simulink model "ArduCopter"  (R2016a)
settings: Solver=ode8  SolverMode=SingleTasking  StartTime=0.0  StopTime=endtime_selfdefine  FixedStep=0.0025  RelTol=1e-3
InitFcn:
  | %load QuadCopterParameters
values from neighbouring files (symbols this model uses):
  Discretetime_400Hz = 0.0025    [euler_roll_angle_cd.mat]
  flight_mode = 1    [flight_control_run.m]
undefined symbols (not defined in the file or in its folder): Cutoff_frequency_acc_z, D_acc_z, D_vel_x, D_vel_y, DEG_TO_RAD, Discretetime_1Hz, g, I_acc_z, I_vel_x, I_vel_y, Kp_angle, MotorLayout, P_acc_z, P_pos_x, P_pos_y, P_pos_z, P_vel_x, P_vel_y, P_vel_z, thrust_rpyt_down, thrust_rpyt_up
libraries: Lib_AC_AttitudeControl x26, Lib_AP_Math x26, Lib_AP_Motors x5, Lib_AC_PID x4, Lib_AP_AHRS x3, simulink x1
(part 1 of 2)
settings Model: Creator=Ehang  LastModifiedBy=Administrator
settings DataIOCC: LimitDataPoints=on  SaveFormat=Array  SaveOutput=off  SaveTime=off
settings DebuggingCC: SignalInfNanChecking=error  SolverPrmCheckMsg=warning  InheritedTsInSrcMsg=none  UnconnectedInputMsg=none  UnconnectedOutputMsg=none  UnconnectedLineMsg=none
settings HardwareCC: ProdBitPerPointer=32  ProdLargestAtomicFloat=None  ProdIntDivRoundTo=Undefined  ProdEndianess=Unspecified  ProdWordSize=32  ProdHWDeviceType=32-bit Generic
settings ModelReferenceCC: ModelReferenceNumInstancesAllowed=Single  PropagateSignalLabelsOutOfModel=off
settings GRTTargetCC: MatFileLogging=off
settings ConfigComp: CovModelRefEnable=Off  CovSFcnEnable=off

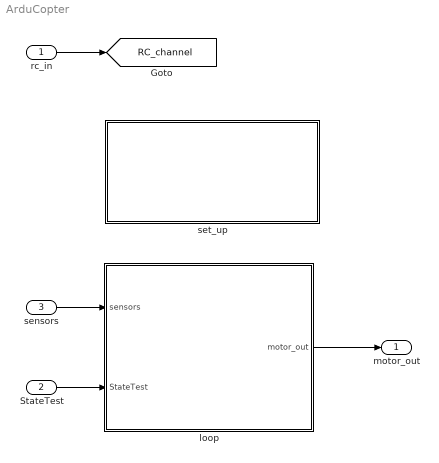
== system ArduCopter ==
  rc_in : Inport  PortDimensions=channelnum
  StateTest : Inport  Port=2  OutDataTypeStr=Bus: VehicleStates
  sensors : Inport  Port=3  OutDataTypeStr=Bus: Sensors
  loop : Subsystem
  set_up : Subsystem  Description=AC_PID控制库
  motor_out : Outport
  tag scope: RC_channel=global
  wires:
  rc_in/1 -> [RC_channel]
  loop/1(motor_out) -> motor_out/1
  sensors/1 -> loop/1(sensors)
  StateTest/1 -> loop/2(StateTest)

== system ArduCopter/loop ==
  sensors : Inport  OutDataTypeStr=Bus: Sensors
  StateTest : Inport  Port=2  OutDataTypeStr=Bus: VehicleStates
  LogData : Subsystem
  Slow-to-Fast Transition1 : RateTransition  OutPortSampleTime=0.0025
  fast_loop : Subsystem
  motors_trysignal : Constant
  scheduler.run : Subsystem  Description=AC_PID控制库
  motor_out : Outport
  wires:
  motors_trysignal/1 -> scheduler.run/1(motors_flag)
  scheduler.run/1(MortorMatix) -> Slow-to-Fast Transition1/1
  Slow-to-Fast Transition1/1 -> fast_loop/3(MotorMatix)
  fast_loop/1(motor_out) -> motor_out/1
  sensors/1 -> fast_loop/1(sensors)
  StateTest/1 -> fast_loop/2(StateTest)

== system ArduCopter/set_up ==

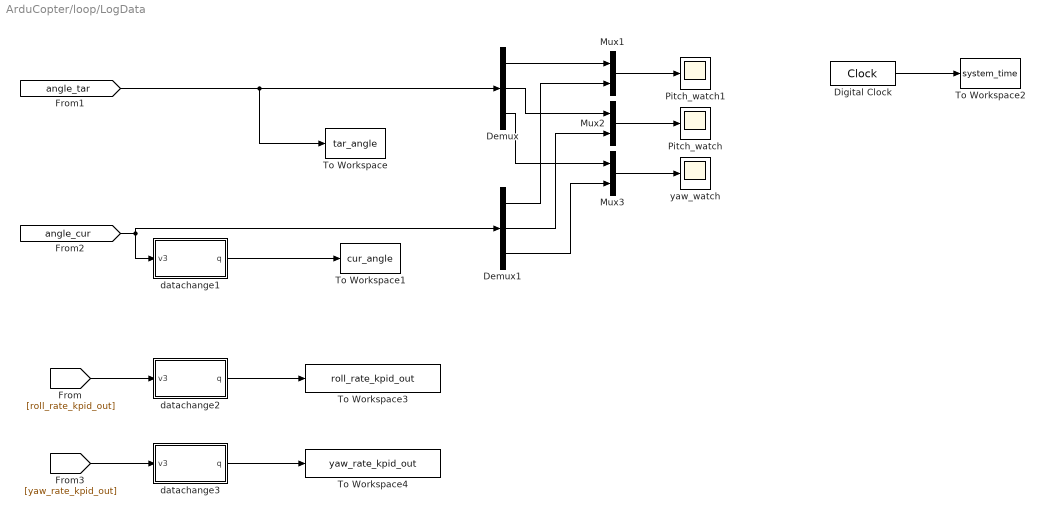
== system ArduCopter/loop/LogData ==
  Demux : Demux  Outputs=3
  Demux1 : Demux  Outputs=3
  Digital Clock : DigitalClock  SampleTime=-1
  Mux1 : Mux  Inputs=2
  Mux2 : Mux  Inputs=2
  Mux3 : Mux  Inputs=2
  Pitch_watch : Scope
  Pitch_watch1 : Scope
  To Workspace : ToWorkspace  VariableName=tar_angle  SaveFormat=Structure  SampleTime=-1
  To Workspace1 : ToWorkspace  VariableName=cur_angle  SaveFormat=Structure  SampleTime=-1
  To Workspace2 : ToWorkspace  VariableName=system_time  SaveFormat=Structure  SampleTime=0.0025
  To Workspace3 : ToWorkspace  VariableName=roll_rate_kpid_out  SaveFormat=Structure  SampleTime=-1
  To Workspace4 : ToWorkspace  VariableName=yaw_rate_kpid_out  SaveFormat=Structure  SampleTime=-1
  datachange1 : MATLAB Function  TreatAsAtomicUnit=on
  datachange2 : MATLAB Function  TreatAsAtomicUnit=on
  datachange3 : MATLAB Function  TreatAsAtomicUnit=on
  yaw_watch : Scope
  wires:
  Mux1/1 -> Pitch_watch1/1
  Demux/1 -> Mux1/1
  Demux1/1 -> Mux1/2
  Mux2/1 -> Pitch_watch/1
  Demux/2 -> Mux2/1
  Demux1/2 -> Mux2/2
  Mux3/1 -> yaw_watch/1
  Demux/3 -> Mux3/1
  Demux1/3 -> Mux3/2
  [angle_tar] -> Demux/1, To Workspace/1
  [roll_rate_kpid_out] -> datachange2/1(v3)
  datachange1/1(q) -> To Workspace1/1
  datachange2/1(q) -> To Workspace3/1
  [angle_cur] -> Demux1/1, datachange1/1(v3)
  Digital Clock/1 -> To Workspace2/1
  [yaw_rate_kpid_out] -> datachange3/1(v3)
  datachange3/1(q) -> To Workspace4/1

== system ArduCopter/loop/fast_loop ==
  sensors : Inport  OutDataTypeStr=Bus: Sensors
  StateTest : Inport  Port=2  OutDataTypeStr=Bus: VehicleStates
  MotorMatix : Inport  Port=3
  AHRS : ModelReference  ModelNameDialog=AHRS  SimulationMode=Normal  ModelReferenceVersion=1.203
  Bus Selector8 : BusSelector  OutputSignals=BodyState.AngularRate
  Mux2 : Mux
  motors_output : Subsystem
  rate_controller_run : Subsystem
  update_flight_mode : Subsystem
  motor_out : Outport
  wires:
  rate_controller_run/1(_roll_in) -> Mux2/2
  rate_controller_run/2(_pitch_in) -> Mux2/3
  rate_controller_run/3(_yaw_in) -> Mux2/4
  update_flight_mode/2(ang_vel_target_rads) -> rate_controller_run/1(ang_vel_target_rads)
  MotorMatix/1 -> motors_output/2(MotorMatix)
  motors_output/1(motor_out) -> motor_out/1
  Mux2/1 -> motors_output/1(thrust)
  sensors/1 -> AHRS/1
  StateTest/1 -> AHRS/2
  AHRS/1 -> Bus Selector8/1, update_flight_mode/1(_ahrs)
  update_flight_mode/1(_throttle_in) -> Mux2/1
  Bus Selector8/1 -> rate_controller_run/2(get_gyro)  "<AngularRate>"

== system ArduCopter/loop/scheduler.run ==
  motors_flag : Inport
  accel_cal_update : Subsystem  Description=AC_PID控制库
  compass_cal_update : Subsystem  Description=AC_PID控制库
  frequence_change : Subsystem
  frequence_change1 : Subsystem
  frequence_change2 : Subsystem
  frequence_change3 : Subsystem
  one_HZ_loop : Subsystem  Description=AC_PID控制库
  ten_hz_logging_loop : Subsystem  Description=AC_PID控制库
  MortorMatix : Outport  PortDimensions=[4,4]
  wires:
  frequence_change/1(Dout) -> one_HZ_loop/1(motors_angle)
  motors_flag/1 -> frequence_change/1(Din), frequence_change1/1(Din), frequence_change2/1(Din), frequence_change3/1(Din)
  frequence_change1/1(Dout) -> ten_hz_logging_loop/1(motors_flag1)
  frequence_change2/1(Dout) -> compass_cal_update/1(motors_flag1)
  frequence_change3/1(Dout) -> accel_cal_update/1(motors_flag1)
  one_HZ_loop/1(MortorMatix) -> MortorMatix/1

== system ArduCopter/loop/fast_loop/motors_output ==
  thrust : Inport  PortDimensions=[4,1]
  MotorMatix : Inport  Port=2
  Display : Display
  motors.output : Subsystem
  motor_out : Outport
  wires:
  thrust/1 -> motors.output/1(thrust)
  MotorMatix/1 -> motors.output/2(MotorMatix)
  motors.output/1(motor_out) -> Display/1, motor_out/1

== system ArduCopter/loop/fast_loop/rate_controller_run ==
  note: roll_sensor
  ang_vel_target_rads : Inport
  get_gyro : Inport  Port=2
  Demux : Demux  Outputs=3
  Demux1 : Demux  Outputs=3  BusSelectionMode=on
  rate_bf_to_motor_pitch : Lib_AC_AttitudeControl/rate_bf_to_motor_pitch
  rate_bf_to_motor_roll : Lib_AC_AttitudeControl/rate_bf_to_motor_roll
  rate_bf_to_motor_yaw : Lib_AC_AttitudeControl/rate_bf_to_motor_yaw
  _roll_in : Outport
  _pitch_in : Outport  Port=2
  _yaw_in : Outport  Port=3
  wires:
  Demux1/3 -> rate_bf_to_motor_yaw/2
  Demux/3 -> rate_bf_to_motor_yaw/1
  rate_bf_to_motor_yaw/1 -> _yaw_in/1
  Demux1/2 -> rate_bf_to_motor_pitch/2
  Demux/2 -> rate_bf_to_motor_pitch/1
  rate_bf_to_motor_pitch/1 -> _pitch_in/1
  Demux1/1 -> rate_bf_to_motor_roll/2
  get_gyro/1 -> Demux1/1
  ang_vel_target_rads/1 -> Demux/1
  rate_bf_to_motor_roll/1 -> _roll_in/1
  Demux/1 -> rate_bf_to_motor_roll/1

== system ArduCopter/loop/fast_loop/update_flight_mode ==
  _ahrs : Inport
  Constant3 : Constant  Value=flight_mode  SampleTime=0.0025
  Multiport Switch : MultiPortSwitch
  Multiport Switch1 : MultiPortSwitch
  althold_run : Subsystem
  poshold_run : Subsystem
  stabilize_run : Subsystem
  _throttle_in : Outport
  ang_vel_target_rads : Outport  Port=2
  wires:
  althold_run/1(_throttle_in) -> Multiport Switch/3
  althold_run/2(ang_vel_target_rads) -> Multiport Switch1/3
  stabilize_run/1(_throttle_in) -> Multiport Switch/2
  stabilize_run/2(ang_vel_target_rads) -> Multiport Switch1/2
  _ahrs/1 -> althold_run/1(_ahrs), poshold_run/1(_ahrs), stabilize_run/1(_ahrs)
  Constant3/1 -> Multiport Switch1/1, Multiport Switch/1
  Multiport Switch1/1 -> ang_vel_target_rads/1
  Multiport Switch/1 -> _throttle_in/1
  poshold_run/1(_throttle_in) -> Multiport Switch/4
  poshold_run/2(ang_vel_target_rads) -> Multiport Switch1/4

== system ArduCopter/loop/scheduler.run/accel_cal_update ==
  motors_flag1 : Inport

== system ArduCopter/loop/scheduler.run/compass_cal_update ==
  motors_flag1 : Inport

== system ArduCopter/loop/scheduler.run/frequence_change ==
  Din : Inport
  Fast-to-Slow Transition1 : RateTransition
  Gain 1 Sample Time: -2 : Gain  SampleTime=0.0025
  Gain 1 Sample Time: -3 : Gain  SampleTime=Discretetime_1Hz
  Slow-to-Fast Transition1 : RateTransition
  Dout : Outport
  wires:
  Slow-to-Fast Transition1/1 -> Gain 1 Sample Time: -2/1
  Gain 1 Sample Time: -2/1 -> Fast-to-Slow Transition1/1
  Fast-to-Slow Transition1/1 -> Gain 1 Sample Time: -3/1
  Gain 1 Sample Time: -3/1 -> Dout/1
  Din/1 -> Slow-to-Fast Transition1/1

== system ArduCopter/loop/scheduler.run/frequence_change1 ==
  Din : Inport
  Fast-to-Slow Transition1 : RateTransition
  Gain 1 Sample Time: -2 : Gain  SampleTime=0.0025
  Gain 1 Sample Time: -3 : Gain  SampleTime=0.1
  Slow-to-Fast Transition1 : RateTransition
  Dout : Outport
  wires:
  Slow-to-Fast Transition1/1 -> Gain 1 Sample Time: -2/1
  Gain 1 Sample Time: -2/1 -> Fast-to-Slow Transition1/1
  Fast-to-Slow Transition1/1 -> Gain 1 Sample Time: -3/1
  Gain 1 Sample Time: -3/1 -> Dout/1
  Din/1 -> Slow-to-Fast Transition1/1

== system ArduCopter/loop/scheduler.run/frequence_change2 ==
  Din : Inport
  Fast-to-Slow Transition1 : RateTransition
  Gain 1 Sample Time: -2 : Gain  SampleTime=0.0025
  Gain 1 Sample Time: -3 : Gain  SampleTime=0.01
  Slow-to-Fast Transition1 : RateTransition
  Dout : Outport
  wires:
  Slow-to-Fast Transition1/1 -> Gain 1 Sample Time: -2/1
  Gain 1 Sample Time: -2/1 -> Fast-to-Slow Transition1/1
  Fast-to-Slow Transition1/1 -> Gain 1 Sample Time: -3/1
  Gain 1 Sample Time: -3/1 -> Dout/1
  Din/1 -> Slow-to-Fast Transition1/1

== system ArduCopter/loop/scheduler.run/frequence_change3 ==
  Din : Inport
  Fast-to-Slow Transition1 : RateTransition
  Gain 1 Sample Time: -2 : Gain  SampleTime=0.0025
  Gain 1 Sample Time: -3 : Gain  SampleTime=0.1
  Slow-to-Fast Transition1 : RateTransition
  Dout : Outport
  wires:
  Slow-to-Fast Transition1/1 -> Gain 1 Sample Time: -2/1
  Gain 1 Sample Time: -2/1 -> Fast-to-Slow Transition1/1
  Fast-to-Slow Transition1/1 -> Gain 1 Sample Time: -3/1
  Gain 1 Sample Time: -3/1 -> Dout/1
  Din/1 -> Slow-to-Fast Transition1/1

== system ArduCopter/loop/scheduler.run/one_HZ_loop ==
  motors_angle : Inport
  set_frame_orientation : Subsystem
  MortorMatix : Outport  PortDimensions=[4,4]
  wires:
  set_frame_orientation/1(MortorMatix) -> MortorMatix/1

== system ArduCopter/loop/scheduler.run/ten_hz_logging_loop ==
  motors_flag1 : Inport

== system ArduCopter/loop/fast_loop/motors_output/motors.output ==
  thrust : Inport
  MotorMatix : Inport  Port=2
  Demux : Demux
  Mux2 : Mux
  output_armed_stabilizing : Subsystem
  output_to_motors : Subsystem
  update_throttle_filter : Subsystem
  motor_out : Outport
  wires:
  MotorMatix/1 -> output_armed_stabilizing/2(MotorMatix)
  output_armed_stabilizing/1(thrust_rpyt_out) -> output_to_motors/1(thrust_rpyt_out)
  output_to_motors/1(motor_out) -> motor_out/1
  update_throttle_filter/1(_throttle_filter.out) -> Mux2/1
  Demux/1 -> update_throttle_filter/1(_throttle_in)
  Demux/2 -> Mux2/2
  Demux/3 -> Mux2/3
  Demux/4 -> Mux2/4
  thrust/1 -> Demux/1
  Mux2/1 -> output_armed_stabilizing/1(thrust)

== system ArduCopter/loop/fast_loop/update_flight_mode/althold_run ==
  _ahrs : Inport
  LoadConstParameter1 : Constant  Value=Discretetime_400Hz  SampleTime=-1
  get_pilot_desired : Subsystem
  input_euler_angle_roll_pitch_euler_rate_yaw_smooth1 : Subsystem
  set_throttle_out : Subsystem
  update_simple_mode : Lib_AC_AttitudeControl/update_simple_mode
  _throttle_in : Outport
  ang_vel_target_rads : Outport  Port=2
  wires:
  get_pilot_desired/2(target_climb_rate) -> set_throttle_out/1(target_climb_rate)
  set_throttle_out/1(_throttle_in1) -> _throttle_in/1
  update_simple_mode/1 -> input_euler_angle_roll_pitch_euler_rate_yaw_smooth1/1(euler_roll_angle_cd)
  _ahrs/1 -> update_simple_mode/2, input_euler_angle_roll_pitch_euler_rate_yaw_smooth1/2(_ahrs), set_throttle_out/2(_ahrs)
  input_euler_angle_roll_pitch_euler_rate_yaw_smooth1/1(ang_vel_target_rads) -> ang_vel_target_rads/1
  LoadConstParameter1/1 -> set_throttle_out/3(dt)
  get_pilot_desired/1(euler_cd) -> update_simple_mode/1

== system ArduCopter/loop/fast_loop/update_flight_mode/poshold_run ==
  _ahrs : Inport
  Demux : Demux  Outputs=3
  LoadConstParameter1 : Constant  Value=Discretetime_400Hz  SampleTime=-1
  get_pilot_desired : Subsystem
  input_euler_angle_roll_pitch_euler_rate_yaw_smooth1 : Subsystem
  pos_controller : Subsystem
  set_throttle_out : Subsystem
  _throttle_in : Outport
  ang_vel_target_rads : Outport  Port=2
  wires:
  set_throttle_out/1(_throttle_in1) -> _throttle_in/1
  _ahrs/1 -> input_euler_angle_roll_pitch_euler_rate_yaw_smooth1/2(_ahrs), pos_controller/5(_ahrs), set_throttle_out/2(_ahrs)
  input_euler_angle_roll_pitch_euler_rate_yaw_smooth1/1(ang_vel_target_rads) -> ang_vel_target_rads/1
  LoadConstParameter1/1 -> pos_controller/4(dt), set_throttle_out/3(dt)
  get_pilot_desired/2(climb_rate_cd) -> set_throttle_out/1(target_climb_rate)
  Demux/1 -> pos_controller/1(velocity_x_cd)
  Demux/2 -> pos_controller/2(velocity_y_cd)
  Demux/3 -> pos_controller/3(yaw_rate_cd)
  get_pilot_desired/1(velocity_cd) -> Demux/1
  pos_controller/1(atitude_des) -> input_euler_angle_roll_pitch_euler_rate_yaw_smooth1/1(euler_roll_angle_cd)

== system ArduCopter/loop/fast_loop/update_flight_mode/stabilize_run ==
  _ahrs : Inport
  get_pilot_desired : Subsystem
  input_euler_angle_roll_pitch_euler_rate_yaw_smooth : Subsystem
  set_throttle_out : Lib_AC_AttitudeControl/set_throttle_out
  update_simple_mode : Lib_AC_AttitudeControl/update_simple_mode
  _throttle_in : Outport
  ang_vel_target_rads : Outport  Port=2
  wires:
  get_pilot_desired/2(pilot_throttle_scaled) -> set_throttle_out/1
  set_throttle_out/1 -> _throttle_in/1
  _ahrs/1 -> update_simple_mode/2, input_euler_angle_roll_pitch_euler_rate_yaw_smooth/2(_ahrs), set_throttle_out/3
  input_euler_angle_roll_pitch_euler_rate_yaw_smooth/1(ang_vel_target_rads) -> ang_vel_target_rads/1
  get_pilot_desired/1(euler_cd) -> update_simple_mode/1
  update_simple_mode/1 -> input_euler_angle_roll_pitch_euler_rate_yaw_smooth/1(euler_roll_angle_cd)

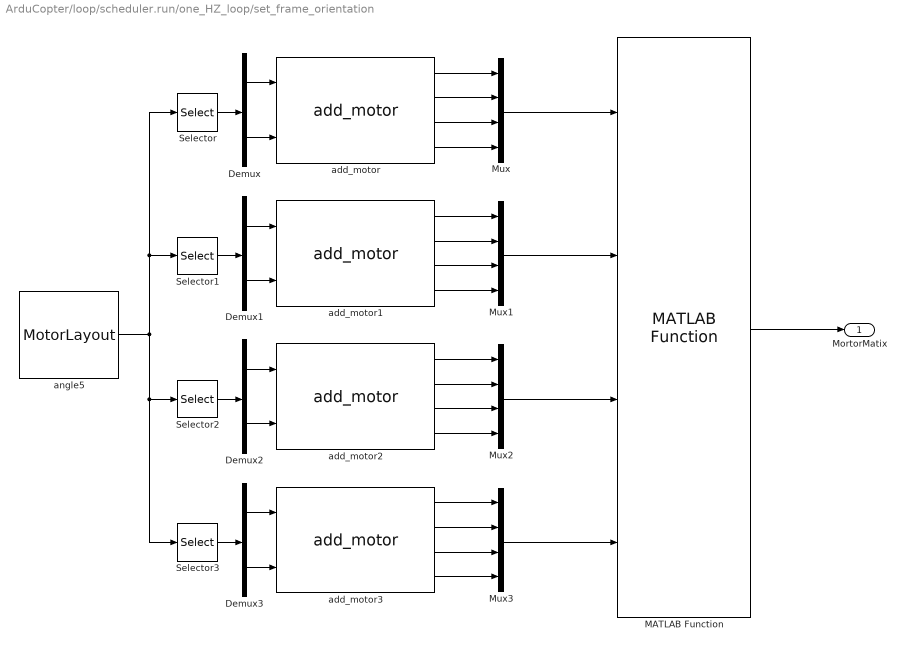
== system ArduCopter/loop/scheduler.run/one_HZ_loop/set_frame_orientation ==
  Demux{,1..3} (4 alike) : Demux  Outputs=2
  MATLAB Function : Lib_AP_Motors/MATLAB Function
  Mux{,1..3} (4 alike) : Mux
  Selector : Selector  NumberOfDimensions=2  InputPortWidth=3  IndexOptions=Index vector (dialog),Index vector (dialog)  Indices=[1],[1 2]  OutputSizes=1,1
  Selector1 : Selector  NumberOfDimensions=2  InputPortWidth=3  IndexOptions=Index vector (dialog),Index vector (dialog)  Indices=[2],[1 2]  OutputSizes=1,1
  Selector2 : Selector  NumberOfDimensions=2  InputPortWidth=3  IndexOptions=Index vector (dialog),Index vector (dialog)  Indices=[3],[1 2]  OutputSizes=1,1
  Selector3 : Selector  NumberOfDimensions=2  InputPortWidth=3  IndexOptions=Index vector (dialog),Index vector (dialog)  Indices=[4],[1 2]  OutputSizes=1,1
  add_motor{,1..3} (4 alike) : Lib_AP_Motors/add_motor
  angle5 : Constant  Description=低通滤波器的时间常数  Value=MotorLayout  SampleTime=Discretetime_1Hz
  MortorMatix : Outport  PortDimensions=[4,4]
  wires:
  add_motor1/4 -> Mux1/4
  add_motor1/2 -> Mux1/2
  add_motor1/3 -> Mux1/3
  add_motor1/1 -> Mux1/1
  Mux1/1 -> MATLAB Function/2
  MATLAB Function/1 -> MortorMatix/1
  add_motor2/2 -> Mux2/2
  add_motor2/3 -> Mux2/3
  add_motor2/4 -> Mux2/4
  Mux2/1 -> MATLAB Function/3
  add_motor2/1 -> Mux2/1
  add_motor/2 -> Mux/2
  Mux/1 -> MATLAB Function/1
  add_motor/3 -> Mux/3
  add_motor/1 -> Mux/1
  add_motor/4 -> Mux/4
  add_motor3/1 -> Mux3/1
  add_motor3/4 -> Mux3/4
  add_motor3/3 -> Mux3/3
  add_motor3/2 -> Mux3/2
  Mux3/1 -> MATLAB Function/4
  Selector/1 -> Demux/1
  Selector1/1 -> Demux1/1
  Selector2/1 -> Demux2/1
  Selector3/1 -> Demux3/1
  angle5/1 -> Selector/1, Selector1/1, Selector3/1, Selector2/1
  Demux/1 -> add_motor/1
  Demux/2 -> add_motor/2
  Demux3/1 -> add_motor3/1
  Demux3/2 -> add_motor3/2
  Demux2/1 -> add_motor2/1
  Demux2/2 -> add_motor2/2
  Demux1/1 -> add_motor1/1
  Demux1/2 -> add_motor1/2

== system ArduCopter/loop/fast_loop/motors_output/motors.output/output_armed_stabilizing ==
  note: 机动角度太大，这就达到了上限制了，角度会振动，注意考虑这个因素，可能使得飞机不稳定。
  thrust : Inport
  MotorMatix : Inport  Port=2
  Constant : Constant  Value=thrust_rpyt_up
  Product : Product  Multiplication=Matrix(*)
  Saturation Dynamic : simulink/Discontinuities/Saturation Dynamic  OutMin=[]  OutMax=[]  OutDataTypeStr=Inherit: Same as second input  OutDataType=fixdt(1, 16)  OutScaling=2^-10  DoSatur=off
  Scope1 : Scope
  throttleMinimum : Constant  Value=thrust_rpyt_down
  thrust_rpyt_out : Outport
  wires:
  MotorMatix/1 -> Product/1
  thrust/1 -> Product/2
  throttleMinimum/1 -> Saturation Dynamic/3
  Constant/1 -> Saturation Dynamic/1
  Product/1 -> Saturation Dynamic/2
  Saturation Dynamic/1 -> Scope1/1, thrust_rpyt_out/1  "rightCommand"

== system ArduCopter/loop/fast_loop/motors_output/motors.output/output_to_motors ==
  thrust_rpyt_out : Inport
  calc_thrust_to_pwm : Subsystem
  motor_out : Outport
  wires:
  thrust_rpyt_out/1 -> calc_thrust_to_pwm/1(thrust_in)
  calc_thrust_to_pwm/1(motor_out) -> motor_out/1

== system ArduCopter/loop/fast_loop/motors_output/motors.output/update_throttle_filter ==
  note: 这里进行了截止频率为0的低筒滤波，等效于1,故省略
  _throttle_in : Inport
  _throttle_filter.out : Outport
  wires:
  _throttle_in/1 -> _throttle_filter.out/1

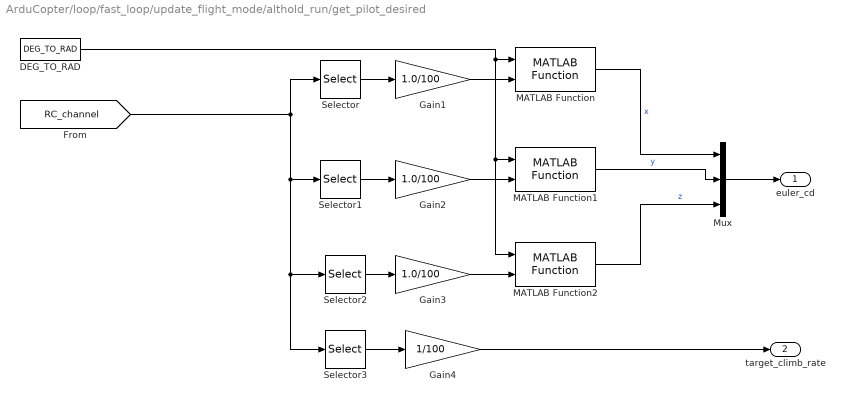
== system ArduCopter/loop/fast_loop/update_flight_mode/althold_run/get_pilot_desired ==
  DEG_TO_RAD : Constant  Description=低通滤波器的时间常数  Value=DEG_TO_RAD
  Gain1 : Gain  Gain=1.0/100
  Gain2 : Gain  Gain=1.0/100
  Gain3 : Gain  Gain=1.0/100
  Gain4 : Gain  Gain=1/100
  MATLAB Function : Lib_AP_Math/MATLAB Function
  MATLAB Function1 : Lib_AP_Math/MATLAB Function
  MATLAB Function2 : Lib_AP_Math/MATLAB Function
  Mux : Mux  Inputs=3
  Selector : Selector  InputPortWidth=6  IndexOptions=Index vector (dialog)  Indices=[1]  OutputSizes=1
  Selector1 : Selector  InputPortWidth=6  IndexOptions=Index vector (dialog)  Indices=[2]  OutputSizes=1
  Selector2 : Selector  InputPortWidth=6  IndexOptions=Index vector (dialog)  Indices=3  OutputSizes=1
  Selector3 : Selector  InputPortWidth=6  IndexOptions=Index vector (dialog)  Indices=4  OutputSizes=1
  euler_cd : Outport
  target_climb_rate : Outport  Port=2
  wires:
  MATLAB Function/1 -> Mux/1  "x"
  MATLAB Function1/1 -> Mux/2  "y"
  MATLAB Function2/1 -> Mux/3  "z"
  Mux/1 -> euler_cd/1
  DEG_TO_RAD/1 -> MATLAB Function/1, MATLAB Function2/1, MATLAB Function1/1
  Selector/1 -> Gain1/1
  Selector1/1 -> Gain2/1
  Selector2/1 -> Gain3/1
  Gain1/1 -> MATLAB Function/2
  Gain2/1 -> MATLAB Function1/2
  Gain3/1 -> MATLAB Function2/2
  Selector3/1 -> Gain4/1
  [RC_channel] -> Selector/1, Selector1/1, Selector2/1, Selector3/1
  Gain4/1 -> target_climb_rate/1

== system ArduCopter/loop/fast_loop/update_flight_mode/althold_run/input_euler_angle_roll_pitch_euler_rate_yaw_smooth1 ==
  euler_roll_angle_cd : Inport
  _ahrs : Inport  Port=2
  MATLAB Function1 : Lib_AC_AttitudeControl/MATLAB Function1
  Subsystem2 : Subsystem
  Unit Delay1 : UnitDelay  InitialCondition=[0 0 0]'  SampleTime=-1
  attitude_controller_run_euler : Subsystem
  ang_vel_target_rads : Outport
  wires:
  Subsystem2/2(att_target_ang_vel_rads) -> MATLAB Function1/2
  Subsystem2/1(Null_att_target_euler_rad_z) -> attitude_controller_run_euler/1(att_target_euler_rad), MATLAB Function1/1
  MATLAB Function1/1 -> attitude_controller_run_euler/2(att_target_ang_vel_rads)
  attitude_controller_run_euler/2(Null_att_target_euler_rad) -> Unit Delay1/1
  Unit Delay1/1 -> Subsystem2/2(Null_att_target_euler_rad)
  euler_roll_angle_cd/1 -> Subsystem2/1(Input_from_rc)
  attitude_controller_run_euler/1(ang_vel_target_rads) -> ang_vel_target_rads/1
  _ahrs/1 -> attitude_controller_run_euler/3(_ahrs)

== system ArduCopter/loop/fast_loop/update_flight_mode/althold_run/set_throttle_out ==
  target_climb_rate : Inport
  _ahrs : Inport  Port=2
  dt : Inport  Port=3
  Scope : Scope  NumInputPorts=3
  Unit Delay : UnitDelay  SampleTime=-1
  set_alt_target_from_climb_rate_ff : Subsystem
  update_z_controller : Subsystem
  _throttle_in1 : Outport
  wires:
  target_climb_rate/1 -> Scope/2, set_alt_target_from_climb_rate_ff/2(climb_rate_cms)
  dt/1 -> set_alt_target_from_climb_rate_ff/3(dt)
  set_alt_target_from_climb_rate_ff/1(Null_pos_target.z) -> Scope/1, Unit Delay/1
  _ahrs/1 -> update_z_controller/2(_ahrs)
  update_z_controller/1(_throttle_in) -> _throttle_in1/1
  Unit Delay/1 -> set_alt_target_from_climb_rate_ff/1(_pos_target.z), update_z_controller/1(_pos_target.z)

== system ArduCopter/loop/fast_loop/update_flight_mode/poshold_run/get_pilot_desired ==
  note: 转为cm/s为单位
  DEG_TO_RAD : Constant  Description=低通滤波器的时间常数  Value=DEG_TO_RAD
  Gain{1..4} (4 alike) : Gain  Gain=1/100
  MATLAB Function2 : Lib_AP_Math/MATLAB Function
  Mux : Mux  Inputs=3
  Selector : Selector  InputPortWidth=6  IndexOptions=Index vector (dialog)  Indices=[1]  OutputSizes=1
  Selector1 : Selector  InputPortWidth=6  IndexOptions=Index vector (dialog)  Indices=[2]  OutputSizes=1
  Selector2 : Selector  InputPortWidth=6  IndexOptions=Index vector (dialog)  Indices=3  OutputSizes=1
  Selector3 : Selector  InputPortWidth=6  IndexOptions=Index vector (dialog)  Indices=4  OutputSizes=1
  velocity_cd : Outport
  climb_rate_cd : Outport  Port=2
  wires:
  Gain1/1 -> Mux/1  "x"
  Gain2/1 -> Mux/2  "y"
  Mux/1 -> velocity_cd/1
  DEG_TO_RAD/1 -> MATLAB Function2/1
  Selector/1 -> Gain1/1
  Selector1/1 -> Gain2/1
  Selector2/1 -> Gain3/1
  Selector3/1 -> Gain4/1
  [RC_channel] -> Selector/1, Selector1/1, Selector2/1, Selector3/1
  Gain3/1 -> MATLAB Function2/2
  MATLAB Function2/1 -> Mux/3  "z"
  Gain4/1 -> climb_rate_cd/1

== system ArduCopter/loop/fast_loop/update_flight_mode/poshold_run/input_euler_angle_roll_pitch_euler_rate_yaw_smooth1 ==
  euler_roll_angle_cd : Inport
  _ahrs : Inport  Port=2
  MATLAB Function1 : Lib_AC_AttitudeControl/MATLAB Function1
  Subsystem2 : Subsystem
  Unit Delay1 : UnitDelay  InitialCondition=[0 0 0]'  SampleTime=-1
  attitude_controller_run_euler : Subsystem
  ang_vel_target_rads : Outport
  wires:
  Subsystem2/2(att_target_ang_vel_rads) -> MATLAB Function1/2
  Subsystem2/1(Null_att_target_euler_rad_z) -> attitude_controller_run_euler/1(att_target_euler_rad), MATLAB Function1/1
  MATLAB Function1/1 -> attitude_controller_run_euler/2(att_target_ang_vel_rads)
  attitude_controller_run_euler/2(Null_att_target_euler_rad) -> Unit Delay1/1
  Unit Delay1/1 -> Subsystem2/2(Null_att_target_euler_rad)
  euler_roll_angle_cd/1 -> Subsystem2/1(Input_from_rc)
  attitude_controller_run_euler/1(ang_vel_target_rads) -> ang_vel_target_rads/1
  _ahrs/1 -> attitude_controller_run_euler/3(_ahrs)

== system ArduCopter/loop/fast_loop/update_flight_mode/poshold_run/pos_controller ==
  velocity_x_cd : Inport
  velocity_y_cd : Inport  Port=2
  yaw_rate_cd : Inport  Port=3
  dt : Inport  Port=4
  _ahrs : Inport  Port=5
  Mux : Mux  Inputs=3
  Saturation : Saturate  UpperLimit=85*pi/180  LowerLimit=-85*pi/180
  Saturation1 : Saturate  UpperLimit=85*pi/180  LowerLimit=-85*pi/180
  calculate_desired_attitude : Subsystem
  pos_to_acc : Subsystem
  pos_to_acc1 : Subsystem
  set_target_pos : Subsystem
  atitude_des : Outport
  wires:
  Mux/1 -> atitude_des/1
  velocity_x_cd/1 -> set_target_pos/1(velocity_x_cd)
  velocity_y_cd/1 -> set_target_pos/2(velocity_y_cd)
  dt/1 -> set_target_pos/3(dt)
  _ahrs/1 -> calculate_desired_attitude/3(_ahrs), pos_to_acc/1(_ahrs), pos_to_acc1/1(_ahrs), set_target_pos/4(_ahrs)
  yaw_rate_cd/1 -> Mux/3
  calculate_desired_attitude/1(roll_des) -> Saturation/1
  pos_to_acc/1(accx_des) -> calculate_desired_attitude/1(accx_des)
  Saturation/1 -> Mux/1
  Saturation1/1 -> Mux/2
  pos_to_acc1/1(accy_des) -> calculate_desired_attitude/2(accy_des)
  calculate_desired_attitude/2(pitch_des) -> Saturation1/1
  set_target_pos/1(pos_tar_x) -> pos_to_acc/2(_pos_target)
  set_target_pos/2(pos_tar_y) -> pos_to_acc1/2(_pos_target)

== system ArduCopter/loop/fast_loop/update_flight_mode/poshold_run/set_throttle_out ==
  target_climb_rate : Inport
  _ahrs : Inport  Port=2
  dt : Inport  Port=3
  Scope : Scope  NumInputPorts=3
  Unit Delay : UnitDelay  SampleTime=-1
  set_alt_target_from_climb_rate_ff : Subsystem
  update_z_controller : Subsystem
  _throttle_in1 : Outport
  wires:
  target_climb_rate/1 -> Scope/2, set_alt_target_from_climb_rate_ff/2(climb_rate_cms)
  dt/1 -> set_alt_target_from_climb_rate_ff/3(dt)
  set_alt_target_from_climb_rate_ff/1(Null_pos_target.z) -> Scope/1, Unit Delay/1
  _ahrs/1 -> update_z_controller/2(_ahrs)
  update_z_controller/1(_throttle_in) -> _throttle_in1/1
  Unit Delay/1 -> set_alt_target_from_climb_rate_ff/1(_pos_target.z), update_z_controller/1(_pos_target.z)

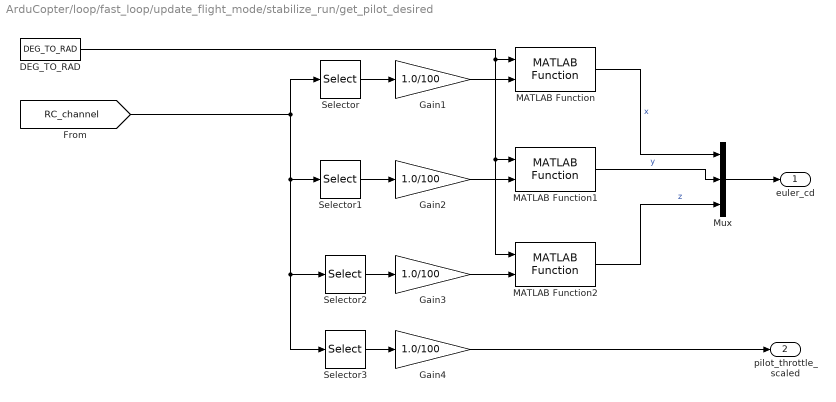
== system ArduCopter/loop/fast_loop/update_flight_mode/stabilize_run/get_pilot_desired ==
  DEG_TO_RAD : Constant  Description=低通滤波器的时间常数  Value=DEG_TO_RAD
  Gain{1..4} (4 alike) : Gain  Gain=1.0/100
  MATLAB Function : Lib_AP_Math/MATLAB Function
  MATLAB Function1 : Lib_AP_Math/MATLAB Function
  MATLAB Function2 : Lib_AP_Math/MATLAB Function
  Mux : Mux  Inputs=3
  Selector : Selector  InputPortWidth=6  IndexOptions=Index vector (dialog)  Indices=[1]  OutputSizes=1
  Selector1 : Selector  InputPortWidth=6  IndexOptions=Index vector (dialog)  Indices=[2]  OutputSizes=1
  Selector2 : Selector  InputPortWidth=6  IndexOptions=Index vector (dialog)  Indices=3  OutputSizes=1
  Selector3 : Selector  InputPortWidth=6  IndexOptions=Index vector (dialog)  Indices=4  OutputSizes=1
  euler_cd : Outport
  pilot_throttle_scaled : Outport  Port=2
  wires:
  MATLAB Function/1 -> Mux/1  "x"
  MATLAB Function1/1 -> Mux/2  "y"
  MATLAB Function2/1 -> Mux/3  "z"
  Mux/1 -> euler_cd/1
  DEG_TO_RAD/1 -> MATLAB Function/1, MATLAB Function2/1, MATLAB Function1/1
  Selector/1 -> Gain1/1
  Selector1/1 -> Gain2/1
  Selector2/1 -> Gain3/1
  Gain1/1 -> MATLAB Function/2
  Gain2/1 -> MATLAB Function1/2
  Gain3/1 -> MATLAB Function2/2
  Selector3/1 -> Gain4/1
  [RC_channel] -> Selector/1, Selector1/1, Selector2/1, Selector3/1
  Gain4/1 -> pilot_throttle_scaled/1

== system ArduCopter/loop/fast_loop/update_flight_mode/stabilize_run/input_euler_angle_roll_pitch_euler_rate_yaw_smooth ==
  euler_roll_angle_cd : Inport
  _ahrs : Inport  Port=2
  MATLAB Function1 : Lib_AC_AttitudeControl/MATLAB Function1
  Subsystem2 : Subsystem
  Unit Delay1 : UnitDelay  InitialCondition=[0 0 0]'  SampleTime=-1
  attitude_controller_run_euler : Subsystem
  ang_vel_target_rads : Outport
  wires:
  Subsystem2/2(att_target_ang_vel_rads) -> MATLAB Function1/2
  Subsystem2/1(Null_att_target_euler_rad_z) -> attitude_controller_run_euler/1(att_target_euler_rad), MATLAB Function1/1
  MATLAB Function1/1 -> attitude_controller_run_euler/2(att_target_ang_vel_rads)
  attitude_controller_run_euler/2(Null_att_target_euler_rad) -> Unit Delay1/1
  Unit Delay1/1 -> Subsystem2/2(Null_att_target_euler_rad)
  euler_roll_angle_cd/1 -> Subsystem2/1(Input_from_rc)
  attitude_controller_run_euler/1(ang_vel_target_rads) -> ang_vel_target_rads/1
  _ahrs/1 -> attitude_controller_run_euler/3(_ahrs)

== system ArduCopter/loop/fast_loop/motors_output/motors.output/output_to_motors/calc_thrust_to_pwm ==
  note: 这个关系是根据输入输出范围简单线性化得到的，有待完善
  thrust_in : Inport
  Add1 : Sum
  Constant : Constant  Value=1100
  Constant1 : Constant  Value=800
  Product : Product
  motor_out : Outport
  wires:
  Constant/1 -> Add1/1
  Constant1/1 -> Product/1
  Product/1 -> Add1/2
  Add1/1 -> motor_out/1
  thrust_in/1 -> Product/2

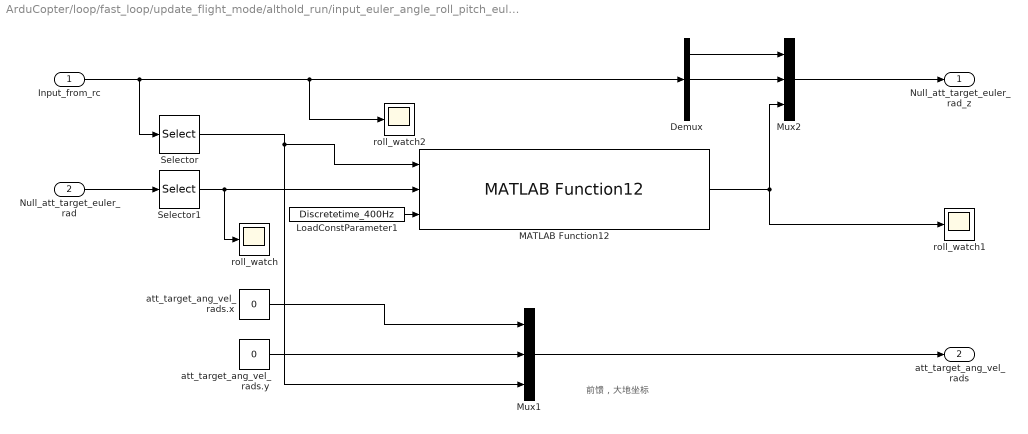
== system ArduCopter/loop/fast_loop/update_flight_mode/althold_run/input_euler_angle_roll_pitch_euler_rate_yaw_smooth1/Subsystem2 ==
  note: 前馈，大地坐标
  Input_from_rc : Inport
  Null_att_target_euler_rad : Inport  Port=2
  Demux : Demux  Outputs=3
  LoadConstParameter1 : Constant  Value=Discretetime_400Hz  SampleTime=-1
  MATLAB Function12 : Lib_AC_AttitudeControl/MATLAB Function12
  Mux1 : Mux  Inputs=3
  Mux2 : Mux  Inputs=3
  Selector : Selector  InputPortWidth=3  IndexOptions=Index vector (dialog)  Indices=[3]  OutputSizes=1
  Selector1 : Selector  InputPortWidth=3  IndexOptions=Index vector (dialog)  Indices=[3]  OutputSizes=1
  att_target_ang_vel_rads.x : Constant  Value=0
  att_target_ang_vel_rads.y : Constant  Value=0
  roll_watch : Scope
  roll_watch1 : Scope
  roll_watch2 : Scope
  Null_att_target_euler_rad_z : Outport
  att_target_ang_vel_rads : Outport  Port=2
  wires:
  Input_from_rc/1 -> Selector/1, Demux/1, roll_watch2/1
  Selector/1 -> MATLAB Function12/1, Mux1/3
  LoadConstParameter1/1 -> MATLAB Function12/3
  MATLAB Function12/1 -> Mux2/3, roll_watch1/1
  Selector1/1 -> MATLAB Function12/2, roll_watch/1
  Null_att_target_euler_rad/1 -> Selector1/1
  Demux/1 -> Mux2/1
  Demux/2 -> Mux2/2
  Mux2/1 -> Null_att_target_euler_rad_z/1
  att_target_ang_vel_rads.x/1 -> Mux1/1
  att_target_ang_vel_rads.y/1 -> Mux1/2
  Mux1/1 -> att_target_ang_vel_rads/1

== system ArduCopter/loop/fast_loop/update_flight_mode/althold_run/input_euler_angle_roll_pitch_euler_rate_yaw_smooth1/attitude_controller_run_euler ==
  att_target_euler_rad : Inport
  att_target_ang_vel_rads : Inport  Port=2
  _ahrs : Inport  Port=3
  Demux : Demux  Outputs=3
  MATLAB Function1 : Lib_AP_Math/MATLAB Function2
  attitude_controller_run_quat : Subsystem
  ang_vel_target_rads : Outport
  Null_att_target_euler_rad : Outport  Port=2
  wires:
  attitude_controller_run_quat/2(Null_att_target_euler_rad) -> Null_att_target_euler_rad/1
  attitude_controller_run_quat/1(ang_vel_target_rads) -> ang_vel_target_rads/1
  att_target_ang_vel_rads/1 -> attitude_controller_run_quat/2(att_target_ang_vel_rads)
  MATLAB Function1/1 -> attitude_controller_run_quat/1(att_target_quat)
  Demux/3 -> MATLAB Function1/3
  Demux/2 -> MATLAB Function1/2
  Demux/1 -> MATLAB Function1/1
  att_target_euler_rad/1 -> Demux/1
  _ahrs/1 -> attitude_controller_run_quat/3(_ahrs)

== system ArduCopter/loop/fast_loop/update_flight_mode/althold_run/set_throttle_out/set_alt_target_from_climb_rate_ff ==
  note: 简化了很多，以后应该补上
  _pos_target.z : Inport
  climb_rate_cms : Inport  Port=2
  dt : Inport  Port=3
  Product : Product
  Subtract : Sum
  Null_pos_target.z : Outport
  wires:
  climb_rate_cms/1 -> Product/1
  dt/1 -> Product/2
  Product/1 -> Subtract/1
  _pos_target.z/1 -> Subtract/2
  Subtract/1 -> Null_pos_target.z/1

== system ArduCopter/loop/fast_loop/update_flight_mode/althold_run/set_throttle_out/update_z_controller ==
  _pos_target.z : Inport
  _ahrs : Inport  Port=2
  pos_to_rate_z : Subsystem
  _throttle_in : Outport
  wires:
  _ahrs/1 -> pos_to_rate_z/1(_ahrs)
  _pos_target.z/1 -> pos_to_rate_z/2(_pos_target.z)
  pos_to_rate_z/1(_throttle_in) -> _throttle_in/1

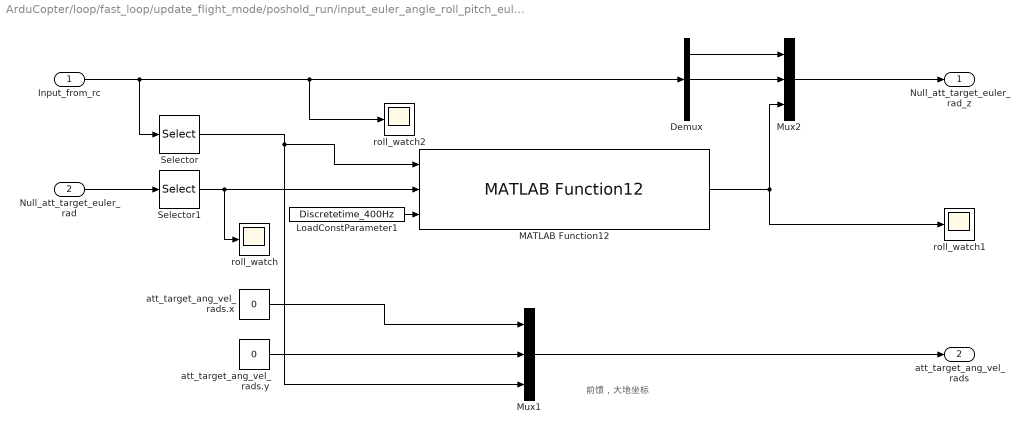
== system ArduCopter/loop/fast_loop/update_flight_mode/poshold_run/input_euler_angle_roll_pitch_euler_rate_yaw_smooth1/Subsystem2 ==
  note: 前馈，大地坐标
  Input_from_rc : Inport
  Null_att_target_euler_rad : Inport  Port=2
  Demux : Demux  Outputs=3
  LoadConstParameter1 : Constant  Value=Discretetime_400Hz  SampleTime=-1
  MATLAB Function12 : Lib_AC_AttitudeControl/MATLAB Function12
  Mux1 : Mux  Inputs=3
  Mux2 : Mux  Inputs=3
  Selector : Selector  InputPortWidth=3  IndexOptions=Index vector (dialog)  Indices=[3]  OutputSizes=1
  Selector1 : Selector  InputPortWidth=3  IndexOptions=Index vector (dialog)  Indices=[3]  OutputSizes=1
  att_target_ang_vel_rads.x : Constant  Value=0
  att_target_ang_vel_rads.y : Constant  Value=0
  roll_watch : Scope
  roll_watch1 : Scope
  roll_watch2 : Scope
  Null_att_target_euler_rad_z : Outport
  att_target_ang_vel_rads : Outport  Port=2
  wires:
  Input_from_rc/1 -> Selector/1, Demux/1, roll_watch2/1
  Selector/1 -> MATLAB Function12/1, Mux1/3
  LoadConstParameter1/1 -> MATLAB Function12/3
  MATLAB Function12/1 -> Mux2/3, roll_watch1/1
  Selector1/1 -> MATLAB Function12/2, roll_watch/1
  Null_att_target_euler_rad/1 -> Selector1/1
  Demux/1 -> Mux2/1
  Demux/2 -> Mux2/2
  Mux2/1 -> Null_att_target_euler_rad_z/1
  att_target_ang_vel_rads.x/1 -> Mux1/1
  att_target_ang_vel_rads.y/1 -> Mux1/2
  Mux1/1 -> att_target_ang_vel_rads/1

== system ArduCopter/loop/fast_loop/update_flight_mode/poshold_run/input_euler_angle_roll_pitch_euler_rate_yaw_smooth1/attitude_controller_run_euler ==
  att_target_euler_rad : Inport
  att_target_ang_vel_rads : Inport  Port=2
  _ahrs : Inport  Port=3
  Demux : Demux  Outputs=3
  MATLAB Function1 : Lib_AP_Math/MATLAB Function2
  attitude_controller_run_quat : Subsystem
  ang_vel_target_rads : Outport
  Null_att_target_euler_rad : Outport  Port=2
  wires:
  attitude_controller_run_quat/2(Null_att_target_euler_rad) -> Null_att_target_euler_rad/1
  attitude_controller_run_quat/1(ang_vel_target_rads) -> ang_vel_target_rads/1
  att_target_ang_vel_rads/1 -> attitude_controller_run_quat/2(att_target_ang_vel_rads)
  MATLAB Function1/1 -> attitude_controller_run_quat/1(att_target_quat)
  Demux/3 -> MATLAB Function1/3
  Demux/2 -> MATLAB Function1/2
  Demux/1 -> MATLAB Function1/1
  att_target_euler_rad/1 -> Demux/1
  _ahrs/1 -> attitude_controller_run_quat/3(_ahrs)

== system ArduCopter/loop/fast_loop/update_flight_mode/poshold_run/pos_controller/calculate_desired_attitude ==
  accx_des : Inport
  accy_des : Inport  Port=2
  _ahrs : Inport  Port=3
  AccMatrix : Constant  Value=[0 1; -1 0]
  Bus Selector : BusSelector  OutputSignals=NEDState.Attitude.Yaw
  Demux : Demux  Outputs=2
  Mux : Mux  Inputs=2
  Product1 : Product  Multiplication=Matrix(*)
  Product2 : Product
  Product3 : Product  Multiplication=Matrix(*)
  c : Constant  Value=1/g(3)
  calculate_Rz_xy : Lib_AC_AttitudeControl/update_simple_mode/calculate_Rz_xy
  roll_des : Outport
  pitch_des : Outport  Port=2
  wires:
  Product1/1 -> Demux/1
  c/1 -> Product2/1
  AccMatrix/1 -> Product2/2
  accx_des/1 -> Mux/1
  accy_des/1 -> Mux/2
  Mux/1 -> Product1/2
  Demux/1 -> roll_des/1
  Demux/2 -> pitch_des/1
  Bus Selector/1 -> calculate_Rz_xy/1  "<Yaw>"
  _ahrs/1 -> Bus Selector/1
  Product2/1 -> Product3/1
  Product3/1 -> Product1/1
  calculate_Rz_xy/1 -> Product3/2

== system ArduCopter/loop/fast_loop/update_flight_mode/poshold_run/pos_controller/pos_to_acc ==
  note: 这应该暂时不用平方根控制器，因为是线性关系
  note: in cm，positive
  _ahrs : Inport
  _pos_target : Inport  Port=2
  Bus Selector : BusSelector  OutputSignals=NEDState.Position.xPos,NEDState.Velocity.xVel
  Gain : Gain  Gain=100
  Gain2 : Gain  Gain=100
  MATLAB Function2 : Lib_AC_AttitudeControl/MATLAB Function2
  Parameter1 : Constant  Value=P_pos_x  SampleTime=-1
  Parameter2 : Constant  Value=250  SampleTime=-1
  Scope : Scope  NumInputPorts=3
  Subtract : Sum  Inputs=+-
  rate_to_accel_z : Subsystem
  accx_des : Outport
  wires:
  _ahrs/1 -> Bus Selector/1
  Bus Selector/1 -> Gain/1  "<xPos>"
  _pos_target/1 -> Scope/1, Subtract/1
  Subtract/1 -> MATLAB Function2/1, Scope/3
  Parameter1/1 -> MATLAB Function2/2
  MATLAB Function2/1 -> rate_to_accel_z/1(_vel_target)
  Gain2/1 -> rate_to_accel_z/2(_vel_cur)
  Bus Selector/2 -> Gain2/1  "<xVel>"
  rate_to_accel_z/1(accx_des) -> accx_des/1
  Gain/1 -> Scope/2, Subtract/2
  Parameter2/1 -> MATLAB Function2/3

== system ArduCopter/loop/fast_loop/update_flight_mode/poshold_run/pos_controller/pos_to_acc1 ==
  note: 这应该暂时不用平方根控制器，因为是线性关系
  note: in cm，positive
  _ahrs : Inport
  _pos_target : Inport  Port=2
  Bus Selector : BusSelector  OutputSignals=NEDState.Position.yPos,NEDState.Velocity.yVel
  Gain : Gain  Gain=100
  Gain2 : Gain  Gain=100
  MATLAB Function2 : Lib_AC_AttitudeControl/MATLAB Function2
  Parameter1 : Constant  Value=P_pos_y  SampleTime=-1
  Parameter2 : Constant  Value=250  SampleTime=-1
  Scope : Scope  NumInputPorts=3
  Subtract : Sum  Inputs=+-
  rate_to_accel_z : Subsystem
  accy_des : Outport
  wires:
  _ahrs/1 -> Bus Selector/1
  Bus Selector/1 -> Gain/1  "<yPos>"
  _pos_target/1 -> Scope/1, Subtract/1
  Subtract/1 -> MATLAB Function2/1, Scope/3
  Parameter1/1 -> MATLAB Function2/2
  MATLAB Function2/1 -> rate_to_accel_z/1(_vel_target)
  Gain2/1 -> rate_to_accel_z/2(_vel_cur)
  Bus Selector/2 -> Gain2/1  "<yVel>"
  rate_to_accel_z/1(accy_des) -> accy_des/1
  Gain/1 -> Scope/2, Subtract/2
  Parameter2/1 -> MATLAB Function2/3

== system ArduCopter/loop/fast_loop/update_flight_mode/poshold_run/pos_controller/set_target_pos ==
  velocity_x_cd : Inport
  velocity_y_cd : Inport  Port=2
  dt : Inport  Port=3
  _ahrs : Inport  Port=4
  Unit Delay : UnitDelay  SampleTime=-1
  Unit Delay1 : UnitDelay  SampleTime=-1
  set_target_from_rate : Subsystem
  set_target_from_rate1 : Subsystem
  update_simple_mode_pos : Lib_AC_AttitudeControl/update_simple_mode_pos
  pos_tar_x : Outport
  pos_tar_y : Outport  Port=2
  wires:
  Unit Delay/1 -> pos_tar_y/1, set_target_from_rate1/1(_pos_target)
  velocity_y_cd/1 -> update_simple_mode_pos/2
  dt/1 -> set_target_from_rate/3(dt), set_target_from_rate1/3(dt)
  set_target_from_rate1/1(Null_pos_target) -> Unit Delay/1
  velocity_x_cd/1 -> update_simple_mode_pos/1
  set_target_from_rate/1(Null_pos_target) -> Unit Delay1/1
  Unit Delay1/1 -> pos_tar_x/1, set_target_from_rate/1(_pos_target)
  _ahrs/1 -> update_simple_mode_pos/3
  update_simple_mode_pos/1 -> set_target_from_rate/2(rate_cms)
  update_simple_mode_pos/2 -> set_target_from_rate1/2(rate_cms)

== system ArduCopter/loop/fast_loop/update_flight_mode/poshold_run/set_throttle_out/set_alt_target_from_climb_rate_ff ==
  note: 简化了很多，以后应该补上
  _pos_target.z : Inport
  climb_rate_cms : Inport  Port=2
  dt : Inport  Port=3
  Product : Product
  Subtract : Sum
  Null_pos_target.z : Outport
  wires:
  climb_rate_cms/1 -> Product/1
  dt/1 -> Product/2
  Product/1 -> Subtract/1
  _pos_target.z/1 -> Subtract/2
  Subtract/1 -> Null_pos_target.z/1

== system ArduCopter/loop/fast_loop/update_flight_mode/poshold_run/set_throttle_out/update_z_controller ==
  _pos_target.z : Inport
  _ahrs : Inport  Port=2
  pos_to_rate_z : Subsystem
  _throttle_in : Outport
  wires:
  _ahrs/1 -> pos_to_rate_z/1(_ahrs)
  _pos_target.z/1 -> pos_to_rate_z/2(_pos_target.z)
  pos_to_rate_z/1(_throttle_in) -> _throttle_in/1

== system ArduCopter/loop/fast_loop/update_flight_mode/stabilize_run/input_euler_angle_roll_pitch_euler_rate_yaw_smooth/Subsystem2 ==
  note: 前馈，大地坐标
  Input_from_rc : Inport
  Null_att_target_euler_rad : Inport  Port=2
  Demux : Demux  Outputs=3
  LoadConstParameter1 : Constant  Value=Discretetime_400Hz  SampleTime=-1
  MATLAB Function12 : Lib_AC_AttitudeControl/MATLAB Function12
  Mux1 : Mux  Inputs=3
  Mux2 : Mux  Inputs=3
  Selector : Selector  InputPortWidth=3  IndexOptions=Index vector (dialog)  Indices=[3]  OutputSizes=1
  Selector1 : Selector  InputPortWidth=3  IndexOptions=Index vector (dialog)  Indices=[3]  OutputSizes=1
  att_target_ang_vel_rads.x : Constant  Value=0
  att_target_ang_vel_rads.y : Constant  Value=0
  roll_watch : Scope
  roll_watch1 : Scope
  roll_watch2 : Scope
  Null_att_target_euler_rad_z : Outport
  att_target_ang_vel_rads : Outport  Port=2
  wires:
  Input_from_rc/1 -> Selector/1, Demux/1, roll_watch2/1
  Selector/1 -> MATLAB Function12/1, Mux1/3
  LoadConstParameter1/1 -> MATLAB Function12/3
  MATLAB Function12/1 -> Mux2/3, roll_watch1/1
  Selector1/1 -> MATLAB Function12/2, roll_watch/1
  Null_att_target_euler_rad/1 -> Selector1/1
  Demux/1 -> Mux2/1
  Demux/2 -> Mux2/2
  Mux2/1 -> Null_att_target_euler_rad_z/1
  att_target_ang_vel_rads.x/1 -> Mux1/1
  att_target_ang_vel_rads.y/1 -> Mux1/2
  Mux1/1 -> att_target_ang_vel_rads/1

== system ArduCopter/loop/fast_loop/update_flight_mode/stabilize_run/input_euler_angle_roll_pitch_euler_rate_yaw_smooth/attitude_controller_run_euler ==
  att_target_euler_rad : Inport
  att_target_ang_vel_rads : Inport  Port=2
  _ahrs : Inport  Port=3
  Bus Selector : BusSelector  OutputSignals=NEDState.Attitude.Roll,NEDState.Attitude.Pitch,NEDState.Attitude.Yaw
  Demux : Demux  Outputs=3
  MATLAB Function1 : Lib_AP_Math/MATLAB Function2
  Mux : Mux  Inputs=3
  Scope1 : Scope
  Scope2 : Scope
  attitude_controller_run_quat : Subsystem
  ang_vel_target_rads : Outport
  Null_att_target_euler_rad : Outport  Port=2
  tag scope: angle_cur=global, angle_tar=global
  wires:
  attitude_controller_run_quat/2(Null_att_target_euler_rad) -> Null_att_target_euler_rad/1
  attitude_controller_run_quat/1(ang_vel_target_rads) -> ang_vel_target_rads/1
  att_target_ang_vel_rads/1 -> attitude_controller_run_quat/2(att_target_ang_vel_rads)
  MATLAB Function1/1 -> attitude_controller_run_quat/1(att_target_quat)
  Demux/3 -> MATLAB Function1/3
  Demux/2 -> MATLAB Function1/2
  Demux/1 -> MATLAB Function1/1
  att_target_euler_rad/1 -> Scope2/1, [angle_tar], Demux/1
  _ahrs/1 -> Bus Selector/1, attitude_controller_run_quat/3(_ahrs)
  Mux/1 -> Scope1/1, [angle_cur]
  Bus Selector/2 -> Mux/2  "<Pitch>"
  Bus Selector/1 -> Mux/1  "<Roll>"
  Bus Selector/3 -> Mux/3  "<Yaw>"

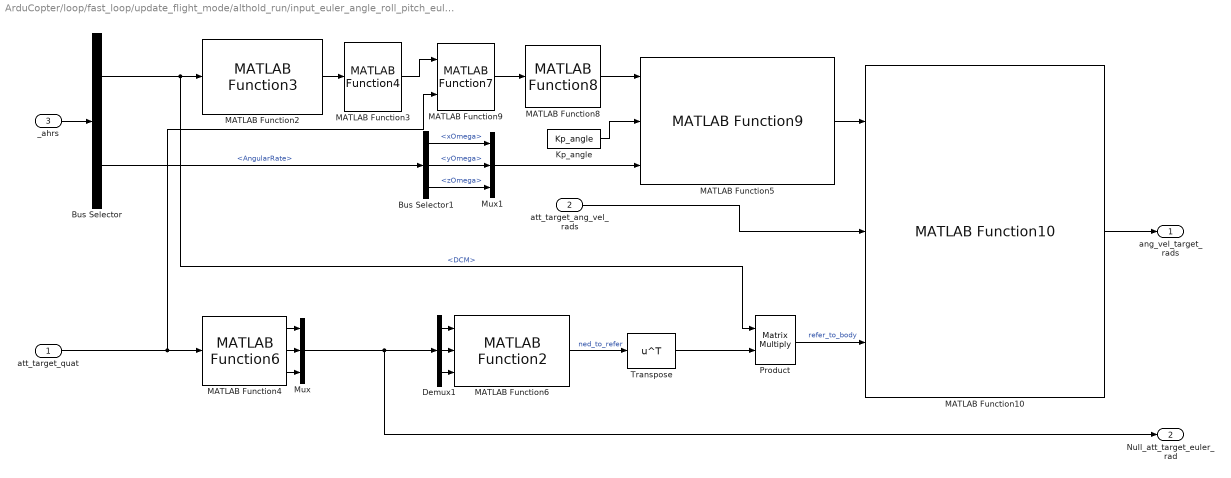
== system ArduCopter/loop/fast_loop/update_flight_mode/althold_run/input_euler_angle_roll_pitch_euler_rate_yaw_smooth1/attitude_controller_run_euler/attitude_controller_run_quat ==
  att_target_quat : Inport
  att_target_ang_vel_rads : Inport  Port=2
  _ahrs : Inport  Port=3
  Bus Selector : BusSelector  OutputSignals=NEDState.Attitude.DCM,BodyState.AngularRate
  Bus Selector1 : BusSelector  OutputSignals=xOmega,yOmega,zOmega
  Demux1 : Demux  Outputs=3
  Kp_angle : Constant  Description=低通滤波器的时间常数  Value=Kp_angle
  MATLAB Function10 : Lib_AC_AttitudeControl/MATLAB Function10
  MATLAB Function2 : Lib_AP_Math/MATLAB Function3
  MATLAB Function3 : Lib_AP_Math/MATLAB Function4
  MATLAB Function4 : Lib_AP_Math/MATLAB Function6
  MATLAB Function5 : Lib_AC_AttitudeControl/MATLAB Function9
  MATLAB Function6 : Lib_AP_AHRS/MATLAB Function2
  MATLAB Function8 : Lib_AP_Math/MATLAB Function8
  MATLAB Function9 : Lib_AP_Math/MATLAB Function7
  Mux : Mux  Inputs=3
  Mux1 : Mux  Inputs=3
  Product : Product  Multiplication=Matrix(*)  RndMeth=Zero
  Transpose : Math  Operator=transpose  SaturateOnIntegerOverflow=on
  ang_vel_target_rads : Outport
  Null_att_target_euler_rad : Outport  Port=2
  wires:
  Mux/1 -> Null_att_target_euler_rad/1, Demux1/1
  MATLAB Function4/1 -> Mux/1
  MATLAB Function4/2 -> Mux/2
  MATLAB Function4/3 -> Mux/3
  MATLAB Function3/1 -> MATLAB Function9/1
  MATLAB Function10/1 -> ang_vel_target_rads/1
  att_target_ang_vel_rads/1 -> MATLAB Function10/2
  MATLAB Function5/1 -> MATLAB Function10/1
  MATLAB Function8/1 -> MATLAB Function5/1
  MATLAB Function9/1 -> MATLAB Function8/1
  MATLAB Function2/1 -> MATLAB Function3/1
  att_target_quat/1 -> MATLAB Function9/2, MATLAB Function4/1
  Kp_angle/1 -> MATLAB Function5/2
  Bus Selector/1 -> Product/1, MATLAB Function2/1  "<DCM>"
  Demux1/1 -> MATLAB Function6/1
  Demux1/2 -> MATLAB Function6/2
  Demux1/3 -> MATLAB Function6/3
  MATLAB Function6/1 -> Transpose/1  "ned_to_refer"
  Transpose/1 -> Product/2
  Product/1 -> MATLAB Function10/3  "refer_to_body"
  _ahrs/1 -> Bus Selector/1
  Bus Selector/2 -> Bus Selector1/1  "<AngularRate>"
  Bus Selector1/2 -> Mux1/2  "<yOmega>"
  Bus Selector1/1 -> Mux1/1  "<xOmega>"
  Bus Selector1/3 -> Mux1/3  "<zOmega>"
  Mux1/1 -> MATLAB Function5/3

== system ArduCopter/loop/fast_loop/update_flight_mode/althold_run/set_throttle_out/update_z_controller/pos_to_rate_z ==
  note: in cm，positive
  _ahrs : Inport
  _pos_target.z : Inport  Port=2
  Bus Selector : BusSelector  OutputSignals=NEDState.Position.zPos,NEDState.Velocity.zVel
  Gain : Gain  Gain=-100
  Gain2 : Gain  Gain=-100
  MATLAB Function1 : Lib_AC_AttitudeControl/MATLAB Function2
  Parameter1 : Constant  Value=P_pos_z  SampleTime=-1
  Parameter2 : Constant  Value=250  SampleTime=-1
  Scope : Scope  NumInputPorts=3
  Subtract : Sum  Inputs=+-
  rate_to_accel_z : Subsystem
  _throttle_in : Outport
  wires:
  _ahrs/1 -> rate_to_accel_z/3(_ahrs), Bus Selector/1
  Bus Selector/1 -> Gain/1  "<zPos>"
  _pos_target.z/1 -> Scope/1, Subtract/1
  Subtract/1 -> MATLAB Function1/1, Scope/3
  Parameter1/1 -> MATLAB Function1/2
  MATLAB Function1/1 -> rate_to_accel_z/1(_vel_target.z)
  Gain2/1 -> rate_to_accel_z/2(_vel_cur.z)
  Bus Selector/2 -> Gain2/1  "<zVel>"
  rate_to_accel_z/1(_throttle_in) -> _throttle_in/1
  Gain/1 -> Scope/2, Subtract/2
  Parameter2/1 -> MATLAB Function1/3

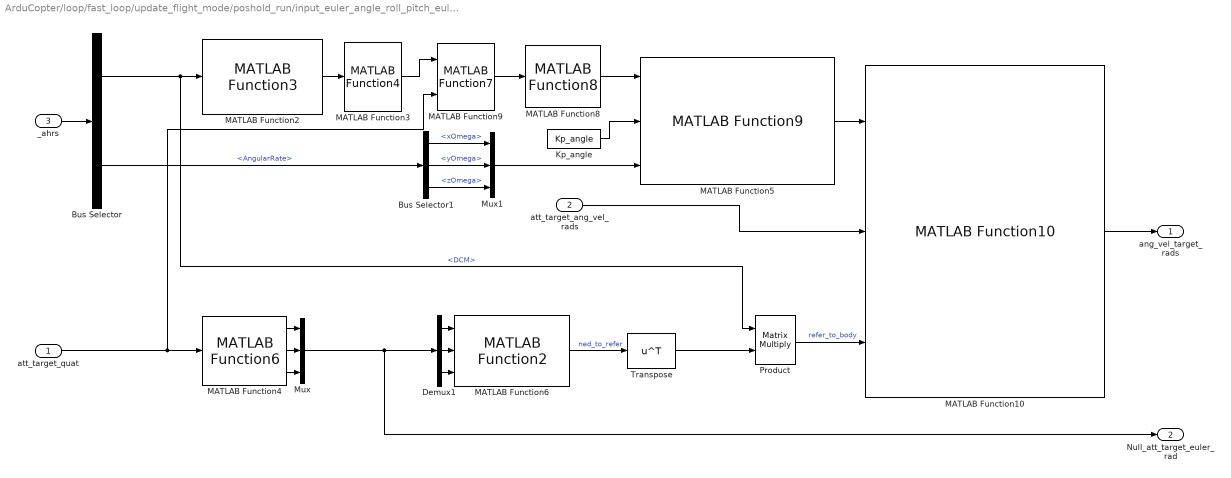
== system ArduCopter/loop/fast_loop/update_flight_mode/poshold_run/input_euler_angle_roll_pitch_euler_rate_yaw_smooth1/attitude_controller_run_euler/attitude_controller_run_quat ==
  att_target_quat : Inport
  att_target_ang_vel_rads : Inport  Port=2
  _ahrs : Inport  Port=3
  Bus Selector : BusSelector  OutputSignals=NEDState.Attitude.DCM,BodyState.AngularRate
  Bus Selector1 : BusSelector  OutputSignals=xOmega,yOmega,zOmega
  Demux1 : Demux  Outputs=3
  Kp_angle : Constant  Description=低通滤波器的时间常数  Value=Kp_angle
  MATLAB Function10 : Lib_AC_AttitudeControl/MATLAB Function10
  MATLAB Function2 : Lib_AP_Math/MATLAB Function3
  MATLAB Function3 : Lib_AP_Math/MATLAB Function4
  MATLAB Function4 : Lib_AP_Math/MATLAB Function6
  MATLAB Function5 : Lib_AC_AttitudeControl/MATLAB Function9
  MATLAB Function6 : Lib_AP_AHRS/MATLAB Function2
  MATLAB Function8 : Lib_AP_Math/MATLAB Function8
  MATLAB Function9 : Lib_AP_Math/MATLAB Function7
  Mux : Mux  Inputs=3
  Mux1 : Mux  Inputs=3
  Product : Product  Multiplication=Matrix(*)  RndMeth=Zero
  Transpose : Math  Operator=transpose  SaturateOnIntegerOverflow=on
  ang_vel_target_rads : Outport
  Null_att_target_euler_rad : Outport  Port=2
  wires:
  Mux/1 -> Null_att_target_euler_rad/1, Demux1/1
  MATLAB Function4/1 -> Mux/1
  MATLAB Function4/2 -> Mux/2
  MATLAB Function4/3 -> Mux/3
  MATLAB Function3/1 -> MATLAB Function9/1
  MATLAB Function10/1 -> ang_vel_target_rads/1
  att_target_ang_vel_rads/1 -> MATLAB Function10/2
  MATLAB Function5/1 -> MATLAB Function10/1
  MATLAB Function8/1 -> MATLAB Function5/1
  MATLAB Function9/1 -> MATLAB Function8/1
  MATLAB Function2/1 -> MATLAB Function3/1
  att_target_quat/1 -> MATLAB Function9/2, MATLAB Function4/1
  Kp_angle/1 -> MATLAB Function5/2
  Bus Selector/1 -> Product/1, MATLAB Function2/1  "<DCM>"
  Demux1/1 -> MATLAB Function6/1
  Demux1/2 -> MATLAB Function6/2
  Demux1/3 -> MATLAB Function6/3
  MATLAB Function6/1 -> Transpose/1  "ned_to_refer"
  Transpose/1 -> Product/2
  Product/1 -> MATLAB Function10/3  "refer_to_body"
  _ahrs/1 -> Bus Selector/1
  Bus Selector/2 -> Bus Selector1/1  "<AngularRate>"
  Bus Selector1/2 -> Mux1/2  "<yOmega>"
  Bus Selector1/1 -> Mux1/1  "<xOmega>"
  Bus Selector1/3 -> Mux1/3  "<zOmega>"
  Mux1/1 -> MATLAB Function5/3

== system ArduCopter/loop/fast_loop/update_flight_mode/poshold_run/pos_controller/pos_to_acc/rate_to_accel_z ==
  _vel_target : Inport
  _vel_cur : Inport  Port=2
  Gain1 : Gain  Gain=1/100  SampleTime=0.0025
  LoadConstParameter1 : Constant  Value=Discretetime_400Hz  SampleTime=-1
  LoadConstParameter5 : Constant  Value=P_vel_x  SampleTime=-1
  LoadConstParameter7 : Constant  Value=D_vel_x  SampleTime=-1
  LoadConstParameter8 : Constant  Value=I_vel_x  SampleTime=-1
  LoadConstParameter9 : Constant  Value=20  SampleTime=-1
  PID_Controller1 : Lib_AC_PID/PID_Controller1  Description=PI控制器。
  Scope : Scope  NumInputPorts=3
  Subtract : Sum  Inputs=+-
  accx_des : Outport
  wires:
  _vel_target/1 -> Scope/1, Subtract/1
  _vel_cur/1 -> Subtract/2, Scope/2
  Subtract/1 -> Scope/3, PID_Controller1/1
  LoadConstParameter5/1 -> PID_Controller1/2
  LoadConstParameter8/1 -> PID_Controller1/3
  LoadConstParameter7/1 -> PID_Controller1/4
  LoadConstParameter9/1 -> PID_Controller1/5
  LoadConstParameter1/1 -> PID_Controller1/6
  PID_Controller1/1 -> Gain1/1
  Gain1/1 -> accx_des/1

== system ArduCopter/loop/fast_loop/update_flight_mode/poshold_run/pos_controller/pos_to_acc1/rate_to_accel_z ==
  _vel_target : Inport
  _vel_cur : Inport  Port=2
  Gain1 : Gain  Gain=1/100  SampleTime=0.0025
  LoadConstParameter1 : Constant  Value=Discretetime_400Hz  SampleTime=-1
  LoadConstParameter5 : Constant  Value=P_vel_y  SampleTime=-1
  LoadConstParameter7 : Constant  Value=D_vel_y  SampleTime=-1
  LoadConstParameter8 : Constant  Value=I_vel_y  SampleTime=-1
  LoadConstParameter9 : Constant  Value=20  SampleTime=-1
  PID_Controller1 : Lib_AC_PID/PID_Controller1  Description=PI控制器。
  Scope : Scope  NumInputPorts=3
  Subtract : Sum  Inputs=+-
  accy_des : Outport
  wires:
  _vel_target/1 -> Scope/1, Subtract/1
  _vel_cur/1 -> Subtract/2, Scope/2
  Subtract/1 -> PID_Controller1/1, Scope/3
  PID_Controller1/1 -> Gain1/1  "_accel_target."
  LoadConstParameter5/1 -> PID_Controller1/2
  LoadConstParameter8/1 -> PID_Controller1/3
  LoadConstParameter7/1 -> PID_Controller1/4
  LoadConstParameter9/1 -> PID_Controller1/5
  LoadConstParameter1/1 -> PID_Controller1/6
  Gain1/1 -> accy_des/1

== system ArduCopter/loop/fast_loop/update_flight_mode/poshold_run/pos_controller/set_target_pos/set_target_from_rate ==
  note: 简化了很多，以后应该补上
  _pos_target : Inport
  rate_cms : Inport  Port=2
  dt : Inport  Port=3
  Product : Product
  Subtract : Sum
  Null_pos_target : Outport
  wires:
  rate_cms/1 -> Product/1
  dt/1 -> Product/2
  Product/1 -> Subtract/1
  _pos_target/1 -> Subtract/2
  Subtract/1 -> Null_pos_target/1

== system ArduCopter/loop/fast_loop/update_flight_mode/poshold_run/pos_controller/set_target_pos/set_target_from_rate1 ==
  note: 简化了很多，以后应该补上
  _pos_target : Inport
  rate_cms : Inport  Port=2
  dt : Inport  Port=3
  Product : Product
  Subtract : Sum
  Null_pos_target : Outport
  wires:
  rate_cms/1 -> Product/1
  dt/1 -> Product/2
  Product/1 -> Subtract/1
  _pos_target/1 -> Subtract/2
  Subtract/1 -> Null_pos_target/1
